simulink model "example_QEKF"  (R2017b)
settings: Solver=FixedStepDiscrete  StartTime=0.0  StopTime=outputs.messages.Time(end)  RelTol=1e-3  EnableMultiTasking=on
InitFcn:
  | CassieModule.importBuses;
values from neighbouring files (symbols this model uses):
  R0 = Lie.Exp(mvnrnd(zeros(3,1),diag(prior_base_pose_std(1:3))^2))    [run.m]
  v0 = mvnrnd(zeros(3,1),diag(prior_base_velocity_std(1:3))^2)    [run.m]
libraries: lib_StateEstimation x4
settings Model: ParamWorkspaceSource=ReferencedWorkspace  Creator=robot  LastModifiedBy=ross
settings DataIOCC: SaveFormat=Array  SaveOutput=off  SignalLogging=off  DSMLogging=off  VisualizeSimOutput=off  SaveTime=off
settings OptimizationCC: DefaultParameterBehavior=Inlined  InlineInvariantSignals=on  LifeSpan=inf  SimCompilerOptimization=on  AccelVerboseBuild=on
settings DebuggingCC: ReadBeforeWriteMsg=DisableAll  WriteAfterWriteMsg=DisableAll  WriteAfterReadMsg=DisableAll  AllowSymbolicDim=off  SFUnexpectedBacktrackingDiag=warning  SFNoUnconditionalDefaultTransitionDiag=warning  SFExecutionAtInitializationDiag=none
settings HardwareCC: ProdBitPerPointer=32  ProdBitPerSizeT=32  ProdBitPerPtrDiffT=32  ProdLargestAtomicFloat=None  ProdWordSize=32  ProdLongLongMode=on  ProdHWDeviceType=Generic->32-bit x86 compatible
settings ModelReferenceCC: UpdateModelReferenceTargets=IfOutOfDate  ParallelModelReferenceMATLABWorkerInit=Copy Base Workspace  ModelReferenceNumInstancesAllowed=Single
settings SFSimCC: SimUserIncludeDirs=gen\kin\src  SFSimEcho=off
settings SFSimCC: SimUserSources=|
  | p_VectorNav_to_RightToeBottom_src.c
  | R_VectorNav_to_RightToeBottom_src.c
  | Jp_VectorNav_to_RightToeBottom_src.c
  | p_VectorNav_to_LeftToeBottom_src.c
  | R_VectorNav_to_LeftToeBottom_src.c
  | Jp_VectorNav_to_LeftToeBottom_src.c
settings RTWCC: SystemTargetFile=slrt.tlc  TLCOptions=-axPCMaxOverloads=1000000000 -axPCMaxOverloadLen=1000000000  TemplateMakefile=slrt_default_tmf  Description=Simulink Real-Time  RTWUseSimCustomCode=on  CustomInclude=gen\kin\src  CodeExecutionProfiling=on  RTWCompilerOptimization=on
settings RTWCC: CustomSource=|
  | p_VectorNav_to_RightToeBottom_src.c
  | R_VectorNav_to_RightToeBottom_src.c
  | Jp_VectorNav_to_RightToeBottom_src.c
  | p_VectorNav_to_LeftToeBottom_src.c
  | R_VectorNav_to_LeftToeBottom_src.c
  | Jp_VectorNav_to_LeftToeBottom_src.c
settings CodeAppCC: GenerateComments=off  MaxIdLength=128  SimulinkBlockComments=off
settings TargetCC: CodeReplacementLibrary=XPC_BLAS  ParMdlRefBuildCompliant=on  ConcurrentExecutionCompliant=on  GeneratePreprocessorConditionals=Use local settings  MatFileLogging=on  MATLABClassNameForMDSCustomization=xpcAperiodicCustomization
settings ConfigComp: CovMetricSettings=dw  CovHtmlReporting=on  CovSaveCumulativeToWorkspaceVar=on  CovSaveSingleToWorkspaceVar=on  CovExternalEMLEnable=off

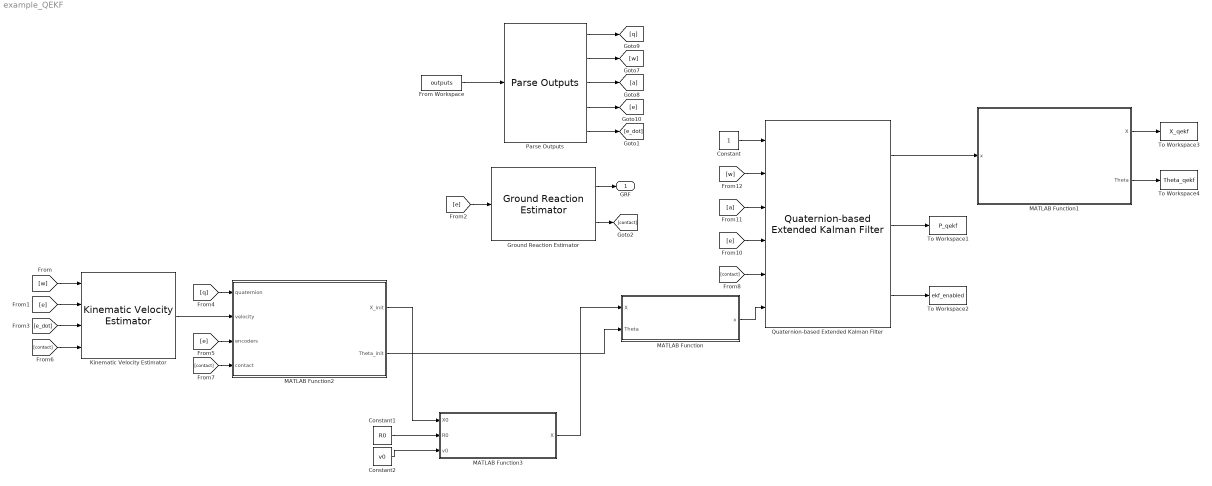
== system example_QEKF ==
  Constant : Constant  SampleTime=-1
  Constant1 : Constant  Value=R0
  Constant2 : Constant  Value=v0
  From Workspace : FromWorkspace  VariableName=outputs  OutDataTypeStr=Bus: CassieOutBus  Interpolate=off  OutputAfterFinalValue=Holding final value
  Ground Reaction Estimator : lib_StateEstimation/Ground Reaction Estimator
  Kinematic Velocity Estimator : lib_StateEstimation/Kinematic Velocity Estimator
  MATLAB Function : MATLAB Function  TreatAsAtomicUnit=on
  MATLAB Function1 : MATLAB Function  TreatAsAtomicUnit=on
  MATLAB Function2 : MATLAB Function  TreatAsAtomicUnit=on
  MATLAB Function3 : MATLAB Function  TreatAsAtomicUnit=on
  Parse Outputs : lib_StateEstimation/Parse Outputs
  Quaternion-based Extended Kalman Filter : lib_StateEstimation/Quaternion-based Extended Kalman Filter
  To Workspace1 : ToWorkspace  VariableName=P_qekf  SaveFormat=Timeseries  SampleTime=-1
  To Workspace2 : ToWorkspace  VariableName=ekf_enabled  SaveFormat=Timeseries  SampleTime=-1
  To Workspace3 : ToWorkspace  VariableName=X_qekf  SaveFormat=Timeseries  SampleTime=-1
  To Workspace4 : ToWorkspace  VariableName=Theta_qekf  SaveFormat=Timeseries  SampleTime=-1
  GRF : Outport
  wires:
  [w] -> Quaternion-based Extended Kalman Filter/2
  [a] -> Quaternion-based Extended Kalman Filter/3
  [e] -> Quaternion-based Extended Kalman Filter/4
  Quaternion-based Extended Kalman Filter/1 -> MATLAB Function1/1(x)
  Quaternion-based Extended Kalman Filter/2 -> To Workspace1/1
  Constant/1 -> Quaternion-based Extended Kalman Filter/1
  MATLAB Function2/1(X_init) -> MATLAB Function3/1(X0)
  Quaternion-based Extended Kalman Filter/3 -> To Workspace2/1
  Parse Outputs/2 -> [w]
  [w] -> Kinematic Velocity Estimator/1
  [e] -> Ground Reaction Estimator/1
  Parse Outputs/3 -> [a]
  Parse Outputs/5 -> [e_dot]
  Ground Reaction Estimator/1 -> GRF/1
  [contact] -> MATLAB Function2/4(contact)
  Kinematic Velocity Estimator/1 -> MATLAB Function2/2(velocity)
  [contact] -> Kinematic Velocity Estimator/4
  [q] -> MATLAB Function2/1(quaternion)
  Ground Reaction Estimator/2 -> [contact]
  [e] -> Kinematic Velocity Estimator/2
  Parse Outputs/4 -> [e]
  [e] -> MATLAB Function2/3(encoders)
  From Workspace/1 -> Parse Outputs/1
  Parse Outputs/1 -> [q]
  [e_dot] -> Kinematic Velocity Estimator/3
  [contact] -> Quaternion-based Extended Kalman Filter/5
  MATLAB Function1/1(X) -> To Workspace3/1
  MATLAB Function1/2(Theta) -> To Workspace4/1
  MATLAB Function2/2(Theta_init) -> MATLAB Function/2(Theta)
  MATLAB Function/1(x) -> Quaternion-based Extended Kalman Filter/6
  Constant2/1 -> MATLAB Function3/3(v0)
  Constant1/1 -> MATLAB Function3/2(R0)
  MATLAB Function3/1(X) -> MATLAB Function/1(X)

== matlab function example_QEKF/MATLAB Function1 ==
  data: x input; X output; Theta output
function [X, Theta]  = ConstructState(x)

Q = Quaternion(x(1:4));
R = Q.getRotation().getValue();
v = x(5:7);
p = x(8:10); 
dL = x(11:13);
dR = x(14:16);
X = eye(7);
X(1:3,:) = [R,v,p,dL,dR];
Theta = x(17:22);

end

== matlab function example_QEKF/MATLAB Function2 ==
  data: quaternion input; velocity input; X_init output; encoders input; contact input; Theta_init output
function [X_init, Theta_init] = InitialStateEstimate(quaternion, velocity, encoders, contact)

% R = Angles.Quaternion_to_Rotation(quaternion);
Q = Quaternion(quaternion);
R = Q.getRotation().getValue();
p = zeros(3,1); 
v = R*velocity;
pR = p_VectorNav_to_RightToeBottom(encoders);
pL = p_VectorNav_to_LeftToeBottom(encoders);

if contact(1) == 1
    % Initialize with left foot at 0
    p = -R * pL; % {W}_p_{WL}
elseif contact(2) == 1
    % Initialize with right foot at 0
    p = -R * pR; % {W}_p_{WR}
end

% Initial foot positions
dL = p + R * pL; % {W}_p_{WL}
dR = p + R * pR; % {W}_p_{WR}

% Construct Initial State
X_init = [R, v, p, dL, dR; 0,0,0,1,0,0,0; 0,0,0,0,1,0,0; 0,0,0,0,0,1,0; 0,0,0,0,0,0,1];

Theta_init = zeros(6,1);

end

== matlab function example_QEKF/MATLAB Function ==
  data: X input; Theta input; x output
function x  = VectorizeState(X, Theta)
R = Rotation3d(X(1:3,1:3));
q = R.getQuaternion.getValue();
x = [q; reshape(X(1:3,4:end),[],1); Theta];
end

== matlab function example_QEKF/MATLAB Function3 ==
  data: X0 input; R0 input; X output; v0 input
function X  = OverwriteState(X0, R0, v0)
X = X0;
X(1:3,1:4) = [R0, v0];
end
